simulink library "PV_lib"  (R2016b)
settings: Solver=ode45  StartTime=0.0  StopTime=10.0  RelTol=1e-3  EnableMultiTasking=on
undefined symbols (not defined in the file): C, D, DiscIntNeverNeededParam, f, I_ki, I_kp, Iac_max, Id_at_max, Iq_at_max, L, PLL_Ki, PLL_Kp, PLL_time_step, Roff, Tau, Td_es_min, Tds, Ts, Vdc_max
libraries: powerlib x42, simulink x16, cstextras x4, powerlib_extras x3, Batt_lib x1, powerlib_meascontrol x1
(part 1 of 2)
settings Model: Creator=re25624  LastModifiedBy=jlesage
settings DataIOCC: LimitDataPoints=on  SaveFormat=Array  SignalLoggingSaveFormat=ModelDataLogs
settings OptimizationCC: ExpressionDepthLimit=2147483647  LifeSpan=inf
settings DebuggingCC: UnderspecifiedInitializationDetection=Classic  MergeDetectMultiDrivingBlocksExec=none  SolverPrmCheckMsg=warning  FcnCallInpInsideContextMsg=warning  StateNameClashWarn=warning  SFUnexpectedBacktrackingDiag=warning  SFNoUnconditionalDefaultTransitionDiag=warning  SFExecutionAtInitializationDiag=none
settings HardwareCC: ProdBitPerPointer=32  ProdBitPerSizeT=32  ProdBitPerPtrDiffT=32  ProdLargestAtomicFloat=None  ProdIntDivRoundTo=Undefined  ProdEndianess=Unspecified  ProdWordSize=32  ProdHWDeviceType=32-bit Generic
settings ModelReferenceCC: PropagateSignalLabelsOutOfModel=off
settings GRTTargetCC: TargetLangStandard=C89/C90 (ANSI)  GeneratePreprocessorConditionals=Disable all  CombineOutputUpdateFcns=off  GRTInterface=on
settings ConfigComp: CovMetricSettings=dw  CovHtmlReporting=on  CovSaveCumulativeToWorkspaceVar=on  CovSaveSingleToWorkspaceVar=on  CovExternalEMLEnable=off

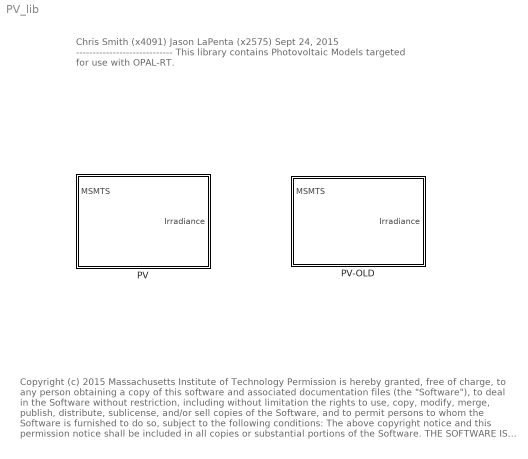
== system PV_lib ==
  note: Chris Smith (x4091)
      | Jason LaPenta (x2575)
      | Sept 24, 2015
      | -----------------------------
      | This library contains Photovoltaic Models
      | targeted for use with OPAL-RT.
  note: Copyright (c) 2015 Massachusetts Institute of Technology
      | Permission is hereby granted, free of charge, to any person obtaining a copy of this software and associated documentation files (the "Software"), to deal in the Software without restriction, including without limitation the rights to use, copy, modify, merge, publish, distribute, sublicense, and/or sell copies of the Software, and to permit persons to whom the Software is furnished to do so, subject to the following conditions:
      |
      | The above copyright notice and this permission notice shall be included in all copies or substantial portions of the Software.
      |
      | THE SOFTWARE IS PROVIDED "AS IS", WITHOUT WARRANTY OF ANY KIND, EXPRESS OR IMPLIED, INCLUDING BUT NOT LIMITED TO THE WARRANTIES OF MERCHANTABILITY, FITNESS FOR A PARTICULAR PURPOSE AND NONINFRINGEMENT. IN NO EVENT SHALL THE AUTHORS OR COPYRIGHT HOLDERS BE LIABLE FOR ANY CLAIM,
      | DAMAGES OR OTHER LIABILITY, WHETHER IN AN ACTION OF CONTRACT, TORT OR OTHERWISE, ARISING FROM, OUT OF OR IN CONNECTION WITH THE SOFTWARE OR THE USE OR OTHER DEALINGS IN THE SOFTWARE.
  PV : Subsystem  mask{max_power=4e6, VacRMS=1200, VacRMS_limit_pu=[1.1 0.9]}
      mask prompts: max_power "Peak Power (W)"; VacRMS "Grid Tie Line to Neutral Voltage (RMS)"; VacRMS_limit_pu "VacRMS Limit [Hi Low] (pu L-N)"
      mask TypeOptions max_power: PV System/max_power
      mask TypeOptions VacRMS: PV System/VacRMS
      mask TypeOptions VacRMS_limit_pu: PV System/VacRMS_limit_pu
  PV-OLD : Subsystem

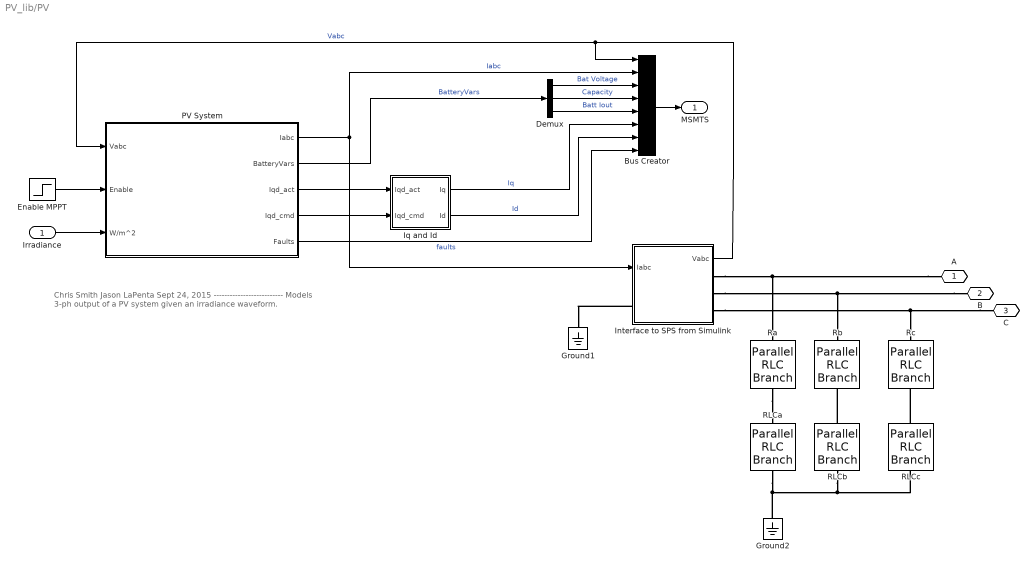
== system PV_lib/PV ==
  note: Chris Smith
      | Jason LaPenta
      | Sept 24, 2015
      | --------------------------
      | Models 3-ph output of a PV system
      | given an irradiance waveform.
  Irradiance : Inport
  Bus Creator : BusCreator  Inputs=8
  Demux : Demux  Outputs=3
  Enable MPPT : Step  Time=0.5  SampleTime=Ts
  Ground1 : powerlib/Elements/Ground  LConnTagsString=a
  Ground2 : powerlib/Elements/Ground  LConnTagsString=a
  Interface to SPS from Simulink : Subsystem
  Iq and Id : Subsystem
  PV System : Subsystem  mask(Battery Energy Storage System with AC inverter and Droop Control){max_power=max_power, VacRMS=VacRMS, Vdc_nom=3500, VacRMS_limit_pu=VacRMS_limit_pu}
      mask prompts: max_power "Peak Power (W)"; VacRMS "Grid Tie Line to Neutral Voltage (RMS)"; Vdc_nom "Nominal DC Battery Voltage"; VacRMS_limit_pu "VacRMS Limit [Hi Low] (pu L-N)"
      mask help: The block implements a battery energy storage system suitable for connecting to the grid. It responds to grid voltage changes by injecting current into the grid. The model is a non-switching average model.
      mask init:
      | %global_parameters
      | BES_init
      mask Help:
      | This block will likely need a filter and transformer on it's output in order to connect to a high power line.
      | 
      | A unit delay block  on the Iabc output can help remove algebraic loops with minimal impact on simulation results.
      | 
      | 
      | Block Parameters:
      | Peak Power- Maximum power the unit can transfer.
      | Capacity- Amount of energy in the battery.
      | Grid Tie Line to Neutral Voltage- RMS voltage for the grid tie interface.
      | Nominal DC Battery Voltage- Open circuit full charge voltage.
      | Real Power Droop Gain- Ratio of Watts to Hz for injecting power to the grid in response to frequency changes.
      | Reactive Power Droop Gain- Ratio of kVars to RMS volts for injecting reactive power to the grid.
      | Droop Filter Cut Off- Fastest frequency that will be responded to for injecting power to the grid.
      | 
      | 
      | Block Connections:
      | Vabc- Grid voltage for each of the three phases.
      | Enable- Set to zero for no power.  Set to 1 to enable energy tranfer.
      | Iabc- Grid current for each of the three phases.  Connect to your grid.  Positive is into the grid.
      | Battery_vars- A vector of battery voltage, capacity, and current out of the battery.
      | Iqd_cmd- Commanded q and d axis currents.
      | Iqd_act- Actual q and d axis currents.
      mask TypeOptions VacRMS_limit_pu: Grid Tied Inverter/VacRMS_limit_pu
  RLCa : powerlib/Elements/Parallel RLC Branch  LConnTagsString=a  RConnTagsString=__new0  BranchType=RLC  Resistance=1e6  Inductance=inf  SetiL0=off  InitialCurrent=0  Capacitance=10e-6  Setx0=off  InitialVoltage=0  Measurements=None
  RLCb : powerlib/Elements/Parallel RLC Branch  LConnTagsString=a  RConnTagsString=__new0  BranchType=RLC  Resistance=1e6  Inductance=inf  SetiL0=off  InitialCurrent=0  Capacitance=10e-6  Setx0=off  InitialVoltage=0  Measurements=None
  "RLCc " : powerlib/Elements/Parallel RLC Branch  LConnTagsString=a  RConnTagsString=__new0  BranchType=RLC  Resistance=1e6  Inductance=inf  SetiL0=off  InitialCurrent=0  Capacitance=10e-6  Setx0=off  InitialVoltage=0  Measurements=None
  Ra : powerlib/Elements/Parallel RLC Branch  LConnTagsString=a  RConnTagsString=__new0  BranchType=R  Resistance=10e-3  Inductance=inf  SetiL0=off  InitialCurrent=0  Capacitance=0  Setx0=off  InitialVoltage=0  Measurements=None
  Rb : powerlib/Elements/Parallel RLC Branch  LConnTagsString=a  RConnTagsString=__new0  BranchType=R  Resistance=10e-3  Inductance=inf  SetiL0=off  InitialCurrent=0  Capacitance=0  Setx0=off  InitialVoltage=0  Measurements=None
  Rc : powerlib/Elements/Parallel RLC Branch  LConnTagsString=a  RConnTagsString=__new0  BranchType=R  Resistance=10e-3  Inductance=inf  SetiL0=off  InitialCurrent=0  Capacitance=0  Setx0=off  InitialVoltage=0  Measurements=None
  A : PMIOPort  Port=1  Side=Right
  B : PMIOPort  Port=2  Side=Right
  C : PMIOPort  Port=3  Side=Right
  MSMTS : Outport
  wires:
  PV System/4(Iqd_cmd) -> Iq and Id/2(Iqd_cmd)
  PV System/5(Faults) -> Bus Creator/8  "faults"
  Enable MPPT/1 -> PV System/2(Enable)
  Bus Creator/1 -> MSMTS/1
  Iq and Id/2(Id) -> Bus Creator/7  "Id"
  PV System/1(Iabc) -> Bus Creator/2, Interface to SPS from Simulink/1(Iabc)  "Iabc"
  Iq and Id/1(Iq) -> Bus Creator/6  "Iq"
  PV System/3(Iqd_act) -> Iq and Id/1(Iqd_act)
  Demux/1 -> Bus Creator/3  "Bat Voltage"
  Demux/3 -> Bus Creator/5  "Batt Iout"
  Demux/2 -> Bus Creator/4  "Capacity"
  PV System/2(BatteryVars) -> Demux/1  "BatteryVars"
  Interface to SPS from Simulink/1(Vabc) -> Bus Creator/1, PV System/1(Vabc)  "Vabc"
  Irradiance/1 -> PV System/3(W/m^2)
  connections:
  Interface to SPS from Simulink/LConn1 -- Ground1/LConn1
  Ra/RConn1 -- RLCa/LConn1
  RLCb/LConn1 -- Rb/RConn1
  "RLCc "/LConn1 -- Rc/RConn1
  A/RConn1 -- Interface to SPS from Simulink/RConn1 -- Ra/LConn1
  C/RConn1 -- Interface to SPS from Simulink/RConn3 -- Rc/LConn1
  B/RConn1 -- Interface to SPS from Simulink/RConn2 -- Rb/LConn1
  "RLCc "/RConn1 -- RLCb/RConn1 -- RLCa/RConn1 -- Ground2/LConn1

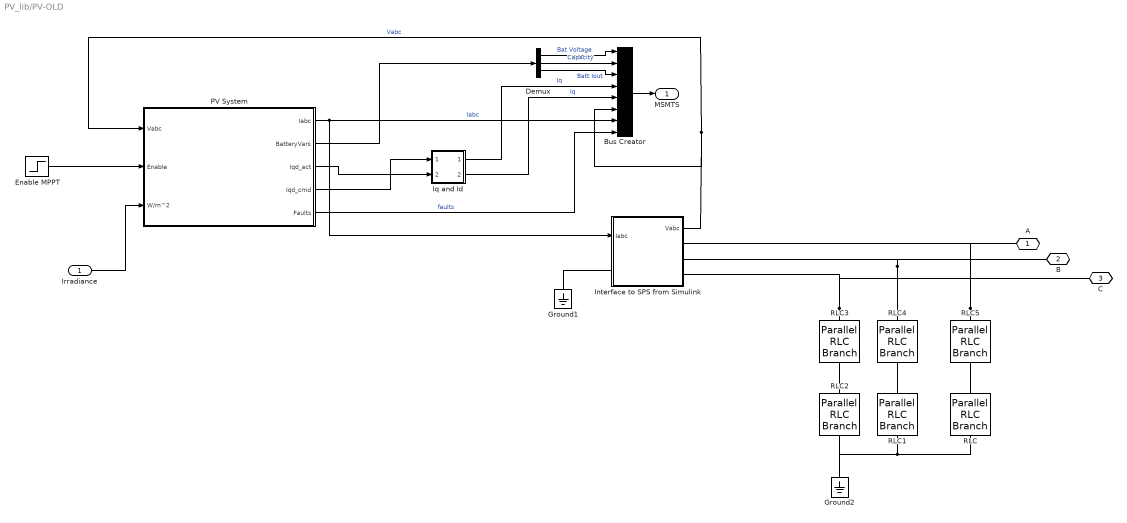
== system PV_lib/PV-OLD ==
  Irradiance : Inport
  Bus Creator : BusCreator  Inputs=8
  Demux : Demux  Outputs=3
  Enable MPPT : Step  Time=0.5  SampleTime=Ts
  Ground1 : powerlib/Elements/Ground  LConnTagsString=a
  Ground2 : powerlib/Elements/Ground  LConnTagsString=a
  Interface to SPS from Simulink : Subsystem
  Iq and Id : Subsystem
  PV System : Subsystem  mask(Battery Energy Storage System with AC inverter and Droop Control){max_power=4e6, VacRMS=1200, Vdc_nom=3500}
      mask prompts: max_power "Peak Power (W)"; VacRMS "Grid Tie Line to Neutral Voltage (RMS)"; Vdc_nom "Nominal DC Battery Voltage"
      mask help: The block implements a battery energy storage system suitable for connecting to the grid. It responds to grid voltage changes by injecting current into the grid. The model is a non-switching average model.
      mask init:
      | global_parameters
      | BES_init
      mask Help:
      | This block will likely need a filter and transformer on it's output in order to connect to a high power line.
      | 
      | A unit delay block  on the Iabc output can help remove algebraic loops with minimal impact on simulation results.
      | 
      | 
      | Block Parameters:
      | Peak Power- Maximum power the unit can transfer.
      | Capacity- Amount of energy in the battery.
      | Grid Tie Line to Neutral Voltage- RMS voltage for the grid tie interface.
      | Nominal DC Battery Voltage- Open circuit full charge voltage.
      | Real Power Droop Gain- Ratio of Watts to Hz for injecting power to the grid in response to frequency changes.
      | Reactive Power Droop Gain- Ratio of kVars to RMS volts for injecting reactive power to the grid.
      | Droop Filter Cut Off- Fastest frequency that will be responded to for injecting power to the grid.
      | 
      | 
      | Block Connections:
      | Vabc- Grid voltage for each of the three phases.
      | Enable- Set to zero for no power.  Set to 1 to enable energy tranfer.
      | Iabc- Grid current for each of the three phases.  Connect to your grid.  Positive is into the grid.
      | Battery_vars- A vector of battery voltage, capacity, and current out of the battery.
      | Iqd_cmd- Commanded q and d axis currents.
      | Iqd_act- Actual q and d axis currents.
  "RLC " : powerlib/Elements/Parallel RLC Branch  LConnTagsString=a  RConnTagsString=__new0  BranchType=RLC  Resistance=1e6  Inductance=inf  SetiL0=off  InitialCurrent=0  Capacitance=10e-6  Setx0=off  InitialVoltage=0  Measurements=None
  RLC1 : powerlib/Elements/Parallel RLC Branch  LConnTagsString=a  RConnTagsString=__new0  BranchType=RLC  Resistance=1e6  Inductance=inf  SetiL0=off  InitialCurrent=0  Capacitance=10e-6  Setx0=off  InitialVoltage=0  Measurements=None
  RLC2 : powerlib/Elements/Parallel RLC Branch  LConnTagsString=a  RConnTagsString=__new0  BranchType=RLC  Resistance=1e6  Inductance=inf  SetiL0=off  InitialCurrent=0  Capacitance=10e-6  Setx0=off  InitialVoltage=0  Measurements=None
  RLC3 : powerlib/Elements/Parallel RLC Branch  LConnTagsString=a  RConnTagsString=__new0  BranchType=R  Resistance=10e-3  Inductance=inf  SetiL0=off  InitialCurrent=0  Capacitance=0  Setx0=off  InitialVoltage=0  Measurements=None
  RLC4 : powerlib/Elements/Parallel RLC Branch  LConnTagsString=a  RConnTagsString=__new0  BranchType=R  Resistance=10e-3  Inductance=inf  SetiL0=off  InitialCurrent=0  Capacitance=0  Setx0=off  InitialVoltage=0  Measurements=None
  RLC5 : powerlib/Elements/Parallel RLC Branch  LConnTagsString=a  RConnTagsString=__new0  BranchType=R  Resistance=10e-3  Inductance=inf  SetiL0=off  InitialCurrent=0  Capacitance=0  Setx0=off  InitialVoltage=0  Measurements=None
  A : PMIOPort  Port=1  Side=Right
  B : PMIOPort  Port=2  Side=Right
  C : PMIOPort  Port=3  Side=Right
  MSMTS : Outport
  wires:
  PV System/4(Iqd_cmd) -> Iq and Id/1(In1)
  PV System/5(Faults) -> Bus Creator/8  "faults"
  Enable MPPT/1 -> PV System/2(Enable)
  Bus Creator/1 -> MSMTS/1
  Iq and Id/2(Out2) -> Bus Creator/5  "Iq"
  PV System/1(Iabc) -> Interface to SPS from Simulink/1(Iabc), Bus Creator/7  "Iabc"
  Iq and Id/1(Out1) -> Bus Creator/4  "Iq"
  PV System/3(Iqd_act) -> Iq and Id/2(In2)
  Demux/1 -> Bus Creator/1  "Bat Voltage"
  Demux/3 -> Bus Creator/3  "Batt Iout"
  Demux/2 -> Bus Creator/2  "Capacity"
  PV System/2(BatteryVars) -> Demux/1
  Interface to SPS from Simulink/1(Vabc) -> PV System/1(Vabc), Bus Creator/6  "Vabc"
  Irradiance/1 -> PV System/3(W/m^2)
  connections:
  "RLC "/LConn1 -- RLC5/RConn1
  RLC1/LConn1 -- RLC4/RConn1
  RLC3/RConn1 -- RLC2/LConn1
  RLC5/LConn1 -- A/RConn1 -- Interface to SPS from Simulink/RConn1
  RLC3/LConn1 -- C/RConn1 -- Interface to SPS from Simulink/RConn3
  Interface to SPS from Simulink/RConn2 -- B/RConn1 -- RLC4/LConn1
  RLC1/RConn1 -- "RLC "/RConn1 -- RLC2/RConn1 -- Ground2/LConn1
  Interface to SPS from Simulink/LConn1 -- Ground1/LConn1

== system PV_lib/PV/Interface to SPS from Simulink ==
  Iabc : Inport
  Demux4 : Demux  Outputs=3
  Gain : Gain  Gain=-1
  Ia : powerlib/Electrical Sources/Controlled Current Source  Initialize=on  Source_Type=AC  Amplitude=0  Phase=0  Frequency=0  Measurements=None
  Ib : powerlib/Electrical Sources/Controlled Current Source  Initialize=on  Source_Type=AC  Amplitude=0  Phase=0  Frequency=0  Measurements=None
  Ic : powerlib/Electrical Sources/Controlled Current Source  Initialize=on  Source_Type=AC  Amplitude=0  Phase=0  Frequency=0  Measurements=None
  Mux2 : Mux  Inputs=3
  Va : powerlib/Measurements/Voltage Measurement  PhasorSimulation=off  OutputType=Complex  PSBequivalent=0
  Vb : powerlib/Measurements/Voltage Measurement  PhasorSimulation=off  OutputType=Complex  PSBequivalent=0
  Vc : powerlib/Measurements/Voltage Measurement  PhasorSimulation=off  OutputType=Complex  PSBequivalent=0
  Phase_A : PMIOPort  Port=1  Side=Right
  Phase_B : PMIOPort  Port=2  Side=Right
  Phase_C : PMIOPort  Port=3  Side=Right
  Ground : PMIOPort  Port=4  Side=Left
  Vabc : Outport
  wires:
  Gain/1 -> Demux4/1
  Va/1 -> Mux2/1
  Mux2/1 -> Vabc/1
  Iabc/1 -> Gain/1
  Demux4/3 -> Ic/1
  Demux4/2 -> Ib/1
  Demux4/1 -> Ia/1
  Vb/1 -> Mux2/2
  Vc/1 -> Mux2/3
  connections:
  Phase_B/RConn1 -- Ib/RConn1 -- Vb/LConn1
  Ground/RConn1 -- Vc/LConn2 -- Va/LConn2 -- Vb/LConn2 -- Ib/LConn1 -- Ia/LConn1 -- Ic/LConn1
  Phase_C/RConn1 -- Ic/RConn1 -- Vc/LConn1
  Ia/RConn1 -- Va/LConn1 -- Phase_A/RConn1

== system PV_lib/PV/Iq and Id ==
  Iqd_act : Inport
  Iqd_cmd : Inport  Port=2
  Demux1 : Demux  Outputs=2
  Demux2 : Demux  Outputs=2
  Mux : Mux  Inputs=2
  Mux1 : Mux  Inputs=2
  Iq : Outport
  Id : Outport  Port=2
  wires:
  Demux1/2 -> Mux1/1  "Id_cmd"
  Demux2/1 -> Mux/2  "Iq_act"
  Demux1/1 -> Mux/1  "Iq_cmd"
  Demux2/2 -> Mux1/2  "Id_act"
  Iqd_cmd/1 -> Demux1/1
  Iqd_act/1 -> Demux2/1
  Mux/1 -> Iq/1
  Mux1/1 -> Id/1

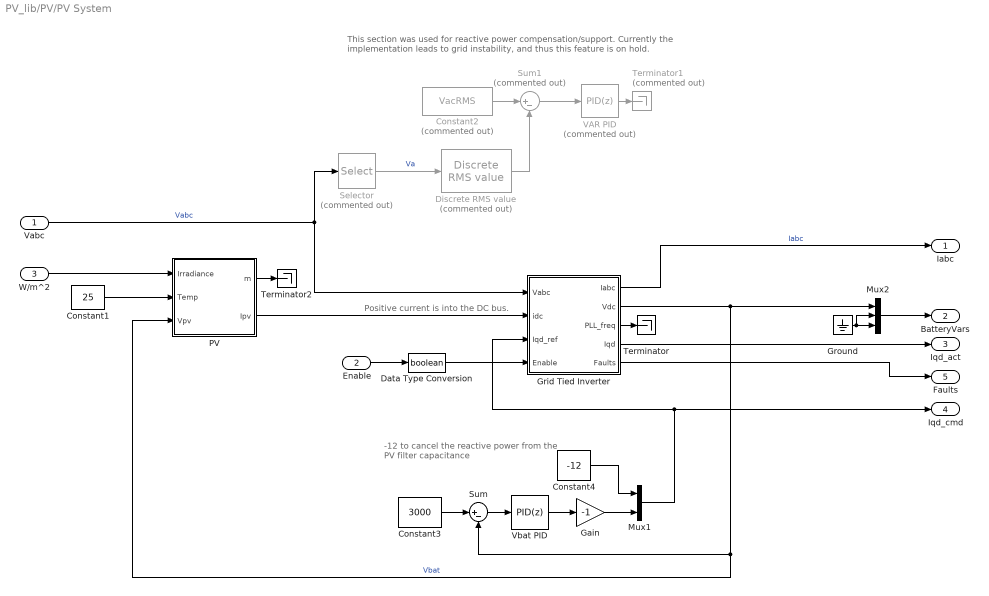
== system PV_lib/PV/PV System ==
  note: Positive current is into the DC bus.
  note: This section was used for reactive power compensation/support.
      | Currently the implementation leads to grid instability, and thus
      | this feature is on hold.
  note: -12 to cancel the reactive power
      | from the PV filter capacitance
  Vabc : Inport
  Enable : Inport  Port=2  OutDataTypeStr=double
  W/m^2 : Inport  Port=3
  Constant1 : Constant  Value=25
  Constant2 : Constant  Commented=on  Value=VacRMS
  Constant3 : Constant  Value=3000
  Constant4 : Constant  Value=-12
  Data Type Conversion : DataTypeConversion  OutDataTypeStr=boolean
  Discrete RMS value : powerlib_extras/Discrete Measurements/Discrete  RMS value  Commented=on  Freq=60  Mag_Init=1200  Ts=Ts
  Gain : Gain  Gain=-1
  Grid Tied Inverter : Subsystem  mask{VacRMS_limit_pu=VacRMS_limit_pu}
      mask prompts: VacRMS_limit_pu "VacRMS Limit [Hi Low] (pu L-N)"
  Ground : Ground
  Mux1 : Mux  Inputs=2
  Mux2 : Mux  Inputs=3
  PV : Subsystem  mask{Ncell=60, Nser=102, Npar=158, Voc_Tref=38, Isc_Tref=8.9, Eg=1.12, dVdI_Voc=-0.32, K0=0.05, Rs=0.349, Rsh=111.55, IL=8.944, Vm=30.5, Im=8.03, PlotVI_module=off, PlotVI_array=off}
      mask prompts: Ncell "Number of cells per module"; Nser "Number of series-connected module per string"; Npar "Numer of parallel strings"; Voc_Tref "Open circuit voltage Voc (V)"; Isc_Tref "Short circuit current Isc (A)"; Eg "Band gap energy of crystalline silicon (eV)"; dVdI_Voc "Temperature coefficient of Voc (%/C)"; K0 "Temperature coefficient of Isc (%/C)"; Rs "Series resistance Rs (Ohms)"; Rsh "Shunt resistance Rsh (Ohms)"; IL "Light-generated current IL (A)"; Vm "Maximum Power Point Voltage Vmpp (V)"; Im "Maximum Powe Point Current Impp (A)"; PlotVI_module "Display  I-V and  P-V characteritics of one module"; PlotVI_array "Display  I-V and  P-V characteritics of array"
      mask init:
      | BlockName=gcb;
      | 
      | 
      | q = 1.6022e-19; % electron charge
      | k = 1.3806e-23; % Boltzman constant
      | n = 1.55; % diode quality factor
      | Tref_K = 273.15+25; % 25C to K
      | Gnom = 1000; % nominal irradiation in W/m^2
      | VT_ref = Ncell*n*k*Tref_K/q; 
      | I0_Tref = Isc_Tref/(exp(Voc_Tref/VT_ref)-1);
      | % Xv = I0_Tref*q*exp(Voc_Tref/VT_ref)/n/k/Tref_K;
      | % Rs = -dVdI_Voc-1/Xv; 
      | 
      | %% Plot I-V & P-V characteristics of one module
      | %==============================================
      | if PlotVI_module | PlotVI_array
      |     assignin('base','Voc_Tref',Voc_Tref);
      |     assignin('base','Isc_Tref',Isc_Tref);
      |     assignin('base','Rs',Rs);
      |     assignin('base','Rsh',Rsh);
      |     assignin('base','I0_Tref',I0_Tref);
      |     assignin('base','VT_ref',VT_ref);
      |      
      |     if PlotVI_module, 
      |         F1 = figure('Name','I-V characteristics of one module at 25 deg.C');
      |         F2 = figure('Name','P-V characteristics of one module at 25 deg.C');
      |     end
      |     if PlotVI_array ,
      |         F3 = figure('Name','I-V characteristics of array at 25 deg.C'); 
      |         F4 = figure('Name','P-V characteristics of array at 25 deg.C'); 
      |     end
      |     load_system('PV_param_plot_model');
      |     
      |     for ksun = 1:-0.2:0.2
      |         assignin('base','IL',IL*ksun)
      |         sim('PV_param_plot_model');
      |         n = find(I_PV >= 0);
      |         I_PV = I_PV(n);
      |         V_PV = V_PV(n);
      |         P_PV = V_PV.*I_PV;
      |         
      |         if PlotVI_module
      |             figure(F1);
      |             if ksun == 1
      |                 
      |                 plot(V_PV,I_PV,'b')
      |                % plot(V_PV,I_PV,'b',[0  Vm Voc_Tref], [Isc_Tref Im 0],'ro')
      |                 text(Voc_Tref/15,Isc_Tref*1.1,'1 kW/m^2')
      |                 hold on
      |                 grid
      |             else
      |                 plot(V_PV,I_PV,'--m')
      |                 text(Voc_Tref/15, Isc_Tref*(ksun+0.1) , sprintf('%g kW/m^2',ksun))
      |             end
      | 
      |             figure(F2); 
      |             if ksun == 1
      |                 
      |                 plot(V_PV,I_PV,'b')
      |                 %plot(V_PV,P_PV,'b',[0  Vm Voc_Tref], [0 Im*Vm 0],'ro')
      |                 text(Vm*1.02,Vm*Im,'1 kW/m^2')
      |                 hold on
      |                 grid
      |             else
      |                 n = find(P_PV == max(P_PV));
      |                 % plot(V_PV,P_PV,'--m', V_PV(n) , P_PV(n),'mo')
      |                 plot(V_PV,P_PV,'--m')
      |                 text(Vm*1.02, Vm*Im*ksun, sprintf('%g kW/m^2',ksun))
      |             end
      |             figure(F1); 
      |             ylabel('Current (A)')
      |             xlabel('Voltage (V)')
      |             axis_xy = axis;
      |             axis_xy(4) = Isc_Tref*1.2;
      |             axis(axis_xy);
      |             
      |             figure(F2);
      |             ylabel('Power (W)')
      |             xlabel('Voltage (V)')
      |             axis_xy = axis;
      |             axis_xy(4) = Vm*Im*1.2;
      |             axis(axis_xy);
      |                   
      |             set_param(BlockName,'PlotVI_module', 'off')
      |         end
      |         
      |         if PlotVI_array
      |             figure(F3);
      |             if ksun == 1
      |                 plot(V_PV*Nser,I_PV*Npar,'b')
      |                 % plot(V_PV*Nser,I_PV*Npar,'b',[0  Vm Voc_Tref]*Nser, [Isc_Tref Im 0]*Npar,'ro')
      |                 text(Voc_Tref/15*Nser,Isc_Tref*1.1*Npar,'1 kW/m^2')
      |                 hold on
      |                 grid
      |             else
      |                 plot(V_PV*Nser,I_PV*Npar,'--m')
      |                 text(Voc_Tref*Nser/15, Isc_Tref*Npar*(ksun+0.1) , sprintf('%g kW/m^2',ksun))
      |             end
      |            
      | 
      |             figure(F4);
      |             if ksun == 1
      |                 plot(V_PV*Nser,P_PV*Nser*Npar,'b')
      |                 % plot(V_PV*Nser,P_PV*Nser*Npar,'b',[0  Vm Voc_Tref]*Nser, [0 Im*Vm 0]*Nser*Npar,'ro')
      |                 text(Vm*Nser*1.02,Vm*Im*Nser*Npar,'1 kW/m^2')
      |                 hold on
      |                 grid
      |             else
      |                 n = find(P_PV == max(P_PV));
      |                 plot(V_PV*Nser,P_PV*Nser*Npar,'--m')
      |                 % plot(V_PV*Nser,P_PV*Nser*Npar,'--m', V_PV(n)*Nser , P_PV(n)*Nser*Npar,'mo')
      |                 text(Vm*Nser*1.02, Vm*Im*Nser*Npar*ksun, sprintf('%g kW/m^2',ksun))
      |             end 
      |             figure(F3);
      |             ylabel('Current (A)')
      |             xlabel('Voltage (V)')
      |             axis_xy = axis;
      |             axis_xy(4) = Isc_Tref*Npar*1.2;
      |             axis(axis_xy);
      |             
      |             figure(F4);
      |             ylabel('Power (W)')
      |             xlabel('Voltage (V)')
      |             xis_xy = axis;
      |             axis_xy(4) = Vm*Im*Nser*Npar*1.2;
      |             axis(axis_xy);
      |             
      |             set_param(BlockName,'PlotVI_array', 'off')
      |         end
      |         
      |     end  
      | end
  Selector : Selector  Commented=on  InputPortWidth=3  IndexOptions=Index vector (dialog)  Indices=[1]  OutputSizes=1
  Sum : Sum  Inputs=|+-
  Sum1 : Sum  Commented=on  Inputs=|+-
  Terminator : Terminator
  Terminator1 : Terminator  Commented=on
  Terminator2 : Terminator
  VAR PID : simulink/Continuous/PID Controller  Commented=on  Controller=PID  TimeDomain=Discrete-time  SampleTime=Ts  IntegratorMethod=Forward Euler  FilterMethod=Forward Euler  Form=Parallel  UseFilter=on  ControllerParametersSource=internal  P=4  I=3  D=0  N=100  InitialConditionSource=internal  InitialConditionForIntegrator=0  InitialConditionForFilter=0  ExternalReset=none  LimitOutput=on  UpperSaturationLimit=2000  LowerSaturationLimit=-2000  LinearizeAsGain=off  AntiWindupMode=clamping  Kb=1  TrackingMode=off  Kt=1  PParamMin=[]  PParamMax=[]  IParamMin=[]  IParamMax=[]  DParamMin=[]  DParamMax=[]  NParamMin=[]  NParamMax=[]  KbParamMin=[]  KbParamMax=[]  KtParamMin=[]  KtParamMax=[]  POutMin=[]  POutMax=[]  IOutMin=[]  IOutMax=[]  DOutMin=[]  DOutMax=[]  NOutMin=[]  NOutMax=[]  KbOutMin=[]  KbOutMax=[]  KtOutMin=[]  KtOutMax=[]  IntegratorOutMin=[]  IntegratorOutMax=[]  FilterOutMin=[]  FilterOutMax=[]  SumOutMin=[]  SumOutMax=[]  SumI1OutMin=[]  SumI1OutMax=[]  SumI2OutMin=[]  SumI2OutMax=[]  SumI3OutMin=[]  SumI3OutMax=[]  SumDOutMin=[]  SumDOutMax=[]  SaturationOutMin=[]  SaturationOutMax=[]  IntegratorContinuousStateAttributes=''  IntegratorStateMustResolveToSignalObject=off  IntegratorRTWStateStorageClass=Auto  FilterContinuousStateAttributes=''  FilterStateMustResolveToSignalObject=off  FilterRTWStateStorageClass=Auto  DifferentiatorICPrevScaledInput=0  DifferentiatorOutMin=[]  DifferentiatorOutMax=[]
  Vbat PID : simulink/Continuous/PID Controller  Controller=PID  TimeDomain=Discrete-time  SampleTime=Ts  IntegratorMethod=Forward Euler  FilterMethod=Forward Euler  Form=Parallel  UseFilter=on  ControllerParametersSource=internal  P=4  I=3  D=0  N=100  InitialConditionSource=internal  InitialConditionForIntegrator=0  InitialConditionForFilter=0  ExternalReset=none  LimitOutput=on  UpperSaturationLimit=2000  LowerSaturationLimit=-2000  LinearizeAsGain=off  AntiWindupMode=clamping  Kb=1  TrackingMode=off  Kt=1  PParamMin=[]  PParamMax=[]  IParamMin=[]  IParamMax=[]  DParamMin=[]  DParamMax=[]  NParamMin=[]  NParamMax=[]  KbParamMin=[]  KbParamMax=[]  KtParamMin=[]  KtParamMax=[]  POutMin=[]  POutMax=[]  IOutMin=[]  IOutMax=[]  DOutMin=[]  DOutMax=[]  NOutMin=[]  NOutMax=[]  KbOutMin=[]  KbOutMax=[]  KtOutMin=[]  KtOutMax=[]  IntegratorOutMin=[]  IntegratorOutMax=[]  FilterOutMin=[]  FilterOutMax=[]  SumOutMin=[]  SumOutMax=[]  SumI1OutMin=[]  SumI1OutMax=[]  SumI2OutMin=[]  SumI2OutMax=[]  SumI3OutMin=[]  SumI3OutMax=[]  SumDOutMin=[]  SumDOutMax=[]  SaturationOutMin=[]  SaturationOutMax=[]  IntegratorContinuousStateAttributes=''  IntegratorStateMustResolveToSignalObject=off  IntegratorRTWStateStorageClass=Auto  FilterContinuousStateAttributes=''  FilterStateMustResolveToSignalObject=off  FilterRTWStateStorageClass=Auto  DifferentiatorICPrevScaledInput=0  DifferentiatorOutMin=[]  DifferentiatorOutMax=[]
  Iabc : Outport
  BatteryVars : Outport  Port=2
  Iqd_act : Outport  Port=3
  Iqd_cmd : Outport  Port=4
  Faults : Outport  Port=5
  wires:
  Grid Tied Inverter/5(Faults) -> Faults/1
  Mux1/1 -> Grid Tied Inverter/3(Iqd_ref), Iqd_cmd/1
  Constant4/1 -> Mux1/1
  Selector/1 -> Discrete RMS value/1  "Va"
  Discrete RMS value/1 -> Sum1/2
  Constant2/1 -> Sum1/1
  Sum1/1 -> VAR PID/1
  Gain/1 -> Mux1/2
  Constant3/1 -> Sum/1
  Vbat PID/1 -> Gain/1
  Sum/1 -> Vbat PID/1
  PV/2(Ipv) -> Grid Tied Inverter/2(idc)
  Constant1/1 -> PV/2(Temp)
  W/m^2/1 -> PV/1(Irradiance)
  Vabc/1 -> Grid Tied Inverter/1(Vabc), Selector/1  "Vabc"
  Grid Tied Inverter/2(Vdc) -> PV/3(Vpv), Sum/2, Mux2/1  "Vbat"
  Grid Tied Inverter/1(Iabc) -> Iabc/1  "Iabc"
  Grid Tied Inverter/4(Iqd) -> Iqd_act/1
  Enable/1 -> Data Type Conversion/1
  Data Type Conversion/1 -> Grid Tied Inverter/4(Enable)
  Mux2/1 -> BatteryVars/1
  Grid Tied Inverter/3(PLL_freq) -> Terminator/1
  VAR PID/1 -> Terminator1/1
  Ground/1 -> Mux2/2, Mux2/3
  PV/1(m) -> Terminator2/1

== system PV_lib/PV-OLD/Interface to SPS from Simulink ==
  Iabc : Inport
  Controlled Current Source3 : powerlib/Electrical Sources/Controlled Current Source  Initialize=on  Source_Type=AC  Amplitude=0  Phase=0  Frequency=0  Measurements=None
  Controlled Current Source4 : powerlib/Electrical Sources/Controlled Current Source  Initialize=on  Source_Type=AC  Amplitude=0  Phase=0  Frequency=0  Measurements=None
  Controlled Current Source5 : powerlib/Electrical Sources/Controlled Current Source  Initialize=on  Source_Type=AC  Amplitude=0  Phase=0  Frequency=0  Measurements=None
  Demux4 : Demux  Outputs=3
  Gain : Gain  Gain=-1
  Mux2 : Mux  Inputs=3
  Voltage Measurement3 : powerlib/Measurements/Voltage Measurement  PhasorSimulation=off  OutputType=Complex  PSBequivalent=0
  Voltage Measurement4 : powerlib/Measurements/Voltage Measurement  PhasorSimulation=off  OutputType=Complex  PSBequivalent=0
  Voltage Measurement5 : powerlib/Measurements/Voltage Measurement  PhasorSimulation=off  OutputType=Complex  PSBequivalent=0
  Phase_A : PMIOPort  Port=1  Side=Right
  Phase_B : PMIOPort  Port=2  Side=Right
  Phase_C : PMIOPort  Port=3  Side=Right
  Ground : PMIOPort  Port=4  Side=Left
  Vabc : Outport
  wires:
  Voltage Measurement5/1 -> Mux2/3
  Voltage Measurement4/1 -> Mux2/2
  Demux4/1 -> Controlled Current Source3/1
  Demux4/2 -> Controlled Current Source4/1
  Demux4/3 -> Controlled Current Source5/1
  Iabc/1 -> Gain/1
  Mux2/1 -> Vabc/1
  Voltage Measurement3/1 -> Mux2/1
  Gain/1 -> Demux4/1
  connections:
  Voltage Measurement5/LConn1 -- Controlled Current Source5/RConn1 -- Phase_C/RConn1
  Voltage Measurement3/LConn1 -- Controlled Current Source3/RConn1 -- Phase_A/RConn1
  Controlled Current Source5/LConn1 -- Controlled Current Source3/LConn1 -- Controlled Current Source4/LConn1 -- Voltage Measurement4/LConn2 -- Voltage Measurement3/LConn2 -- Voltage Measurement5/LConn2 -- Ground/RConn1
  Voltage Measurement4/LConn1 -- Controlled Current Source4/RConn1 -- Phase_B/RConn1

== system PV_lib/PV-OLD/Iq and Id ==
  In1 : Inport
  In2 : Inport  Port=2
  Demux1 : Demux  Outputs=2
  Demux2 : Demux  Outputs=2
  Mux : Mux  Inputs=2
  Mux1 : Mux  Inputs=2
  Out1 : Outport
  Out2 : Outport  Port=2
  wires:
  Mux1/1 -> Out2/1
  Mux/1 -> Out1/1
  In2/1 -> Demux2/1
  In1/1 -> Demux1/1
  Demux2/2 -> Mux1/2  "Id_act"
  Demux1/1 -> Mux/1  "Iq_cmd"
  Demux2/1 -> Mux/2  "Iq_act"
  Demux1/2 -> Mux1/1  "Id_cmd"

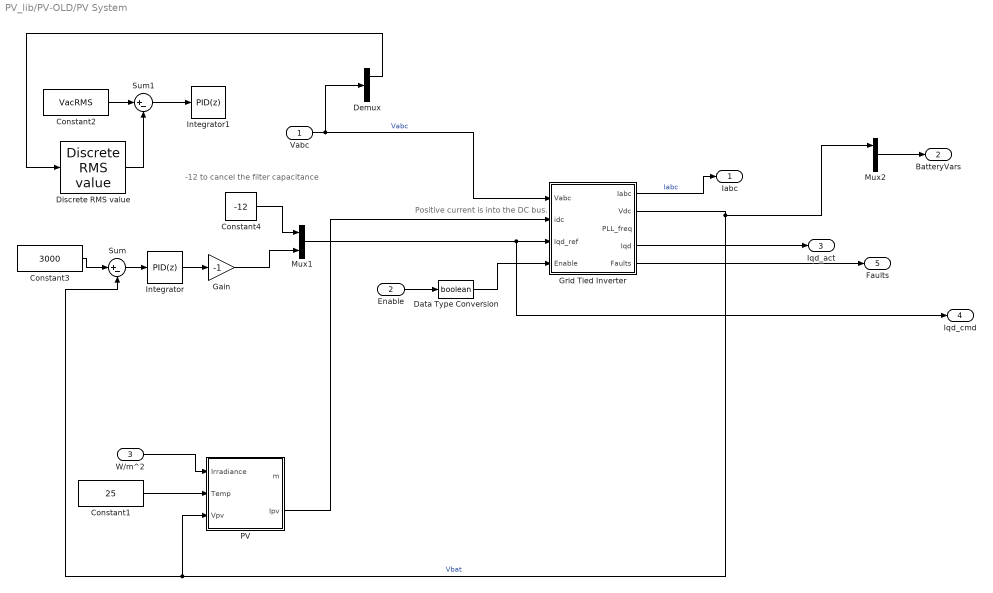
== system PV_lib/PV-OLD/PV System ==
  note: Positive current is into the DC bus.
  note: -12 to cancel the filter capacitance
  Vabc : Inport
  Enable : Inport  Port=2  OutDataTypeStr=double
  W/m^2 : Inport  Port=3
  Constant1 : Constant  Value=25
  Constant2 : Constant  Value=VacRMS
  Constant3 : Constant  Value=3000
  Constant4 : Constant  Value=-12
  Data Type Conversion : DataTypeConversion  OutDataTypeStr=boolean
  Demux : Demux  Outputs=3
  Discrete RMS value : powerlib_extras/Discrete Measurements/Discrete  RMS value  Freq=60  Mag_Init=1200  Ts=Ts
  Gain : Gain  Gain=-1
  Grid Tied Inverter : Subsystem
  Integrator : simulink/Continuous/PID Controller  Controller=PID  TimeDomain=Discrete-time  SampleTime=Ts  IntegratorMethod=Forward Euler  FilterMethod=Forward Euler  Form=Parallel  UseFilter=on  ControllerParametersSource=internal  P=4  I=3  D=0  N=100  InitialConditionSource=internal  InitialConditionForIntegrator=0  InitialConditionForFilter=0  ExternalReset=none  LimitOutput=on  UpperSaturationLimit=2000  LowerSaturationLimit=-2000  LinearizeAsGain=off  AntiWindupMode=clamping  Kb=1  TrackingMode=off  Kt=1  PParamMin=[]  PParamMax=[]  IParamMin=[]  IParamMax=[]  DParamMin=[]  DParamMax=[]  NParamMin=[]  NParamMax=[]  KbParamMin=[]  KbParamMax=[]  KtParamMin=[]  KtParamMax=[]  POutMin=[]  POutMax=[]  IOutMin=[]  IOutMax=[]  DOutMin=[]  DOutMax=[]  NOutMin=[]  NOutMax=[]  KbOutMin=[]  KbOutMax=[]  KtOutMin=[]  KtOutMax=[]  IntegratorOutMin=[]  IntegratorOutMax=[]  FilterOutMin=[]  FilterOutMax=[]  SumOutMin=[]  SumOutMax=[]  SumI1OutMin=[]  SumI1OutMax=[]  SumI2OutMin=[]  SumI2OutMax=[]  SumI3OutMin=[]  SumI3OutMax=[]  SumDOutMin=[]  SumDOutMax=[]  SaturationOutMin=[]  SaturationOutMax=[]  IntegratorContinuousStateAttributes=''  IntegratorStateMustResolveToSignalObject=off  IntegratorRTWStateStorageClass=Auto  FilterContinuousStateAttributes=''  FilterStateMustResolveToSignalObject=off  FilterRTWStateStorageClass=Auto  DifferentiatorICPrevScaledInput=0  DifferentiatorOutMin=[]  DifferentiatorOutMax=[]
  Integrator1 : simulink/Continuous/PID Controller  Controller=PID  TimeDomain=Discrete-time  SampleTime=Ts  IntegratorMethod=Forward Euler  FilterMethod=Forward Euler  Form=Parallel  UseFilter=on  ControllerParametersSource=internal  P=4  I=3  D=0  N=100  InitialConditionSource=internal  InitialConditionForIntegrator=0  InitialConditionForFilter=0  ExternalReset=none  LimitOutput=on  UpperSaturationLimit=2000  LowerSaturationLimit=-2000  LinearizeAsGain=off  AntiWindupMode=clamping  Kb=1  TrackingMode=off  Kt=1  PParamMin=[]  PParamMax=[]  IParamMin=[]  IParamMax=[]  DParamMin=[]  DParamMax=[]  NParamMin=[]  NParamMax=[]  KbParamMin=[]  KbParamMax=[]  KtParamMin=[]  KtParamMax=[]  POutMin=[]  POutMax=[]  IOutMin=[]  IOutMax=[]  DOutMin=[]  DOutMax=[]  NOutMin=[]  NOutMax=[]  KbOutMin=[]  KbOutMax=[]  KtOutMin=[]  KtOutMax=[]  IntegratorOutMin=[]  IntegratorOutMax=[]  FilterOutMin=[]  FilterOutMax=[]  SumOutMin=[]  SumOutMax=[]  SumI1OutMin=[]  SumI1OutMax=[]  SumI2OutMin=[]  SumI2OutMax=[]  SumI3OutMin=[]  SumI3OutMax=[]  SumDOutMin=[]  SumDOutMax=[]  SaturationOutMin=[]  SaturationOutMax=[]  IntegratorContinuousStateAttributes=''  IntegratorStateMustResolveToSignalObject=off  IntegratorRTWStateStorageClass=Auto  FilterContinuousStateAttributes=''  FilterStateMustResolveToSignalObject=off  FilterRTWStateStorageClass=Auto  DifferentiatorICPrevScaledInput=0  DifferentiatorOutMin=[]  DifferentiatorOutMax=[]
  Mux1 : Mux  Inputs=2
  Mux2 : Mux  Inputs=3
  PV : Subsystem  mask{Ncell=60, Nser=102, Npar=158, Voc_Tref=38, Isc_Tref=8.9, Eg=1.12, dVdI_Voc=-0.32, K0=0.05, Rs=0.349, Rsh=111.55, IL=8.944, Vm=30.5, Im=8.03, PlotVI_module=off, PlotVI_array=off}
      mask prompts: Ncell "Number of cells per module"; Nser "Number of series-connected module per string"; Npar "Numer of parallel strings"; Voc_Tref "Open circuit voltage Voc (V)"; Isc_Tref "Short circuit current Isc (A)"; Eg "Band gap energy of crystalline silicon (eV)"; dVdI_Voc "Temperature coefficient of Voc (%/C)"; K0 "Temperature coefficient of Isc (%/C)"; Rs "Series resistance Rs (Ohms)"; Rsh "Shunt resistance Rsh (Ohms)"; IL "Light-generated current IL (A)"; Vm "Maximum Power Point Voltage Vmpp (V)"; Im "Maximum Powe Point Current Impp (A)"; PlotVI_module "Display  I-V and  P-V characteritics of one module"; PlotVI_array "Display  I-V and  P-V characteritics of array"
      mask init: same as PV_lib/PV/PV System/PV
  Sum : Sum  Inputs=|+-
  Sum1 : Sum  Inputs=|+-
  Iabc : Outport
  BatteryVars : Outport  Port=2
  Iqd_act : Outport  Port=3
  Iqd_cmd : Outport  Port=4
  Faults : Outport  Port=5
  wires:
  Mux2/1 -> BatteryVars/1
  Data Type Conversion/1 -> Grid Tied Inverter/4(Enable)
  Enable/1 -> Data Type Conversion/1
  Grid Tied Inverter/4(Iqd) -> Iqd_act/1
  Grid Tied Inverter/1(Iabc) -> Iabc/1  "Iabc"
  Grid Tied Inverter/2(Vdc) -> Mux2/1, PV/3(Vpv), Sum/2  "Vbat"
  Vabc/1 -> Grid Tied Inverter/1(Vabc), Demux/1  "Vabc"
  W/m^2/1 -> PV/1(Irradiance)
  Constant1/1 -> PV/2(Temp)
  PV/2(Ipv) -> Grid Tied Inverter/2(idc)
  Mux1/1 -> Grid Tied Inverter/3(Iqd_ref), Iqd_cmd/1
  Sum/1 -> Integrator/1
  Integrator/1 -> Gain/1
  Constant3/1 -> Sum/1
  Gain/1 -> Mux1/2
  Sum1/1 -> Integrator1/1
  Constant2/1 -> Sum1/1
  Discrete RMS value/1 -> Sum1/2
  Demux/1 -> Discrete RMS value/1
  Grid Tied Inverter/5(Faults) -> Faults/1
  Constant4/1 -> Mux1/1

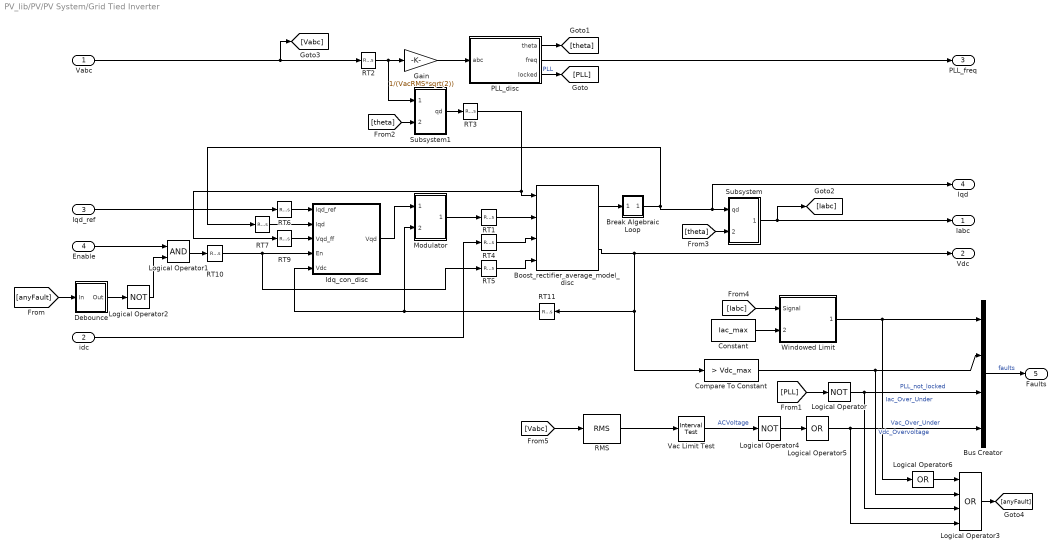
== system PV_lib/PV/PV System/Grid Tied Inverter ==
  Vabc : Inport
  idc : Inport  Port=2
  Iqd_ref : Inport  Port=3
  Enable : Inport  Port=4
  Boost_rectifier_average_model_disc : Batt_lib/HIL_BATT/Batt/Grid Tied Inverter/Boost_rectifier_average_model_disc  C=C  L=L  Roff=Roff  Vdc_nom=Vdc_nom
  Break Algebraic Loop : Subsystem  mask{Tau=Tau, Ts=Ts}
      mask prompts: Tau "Time Constant"; Ts "Sample Time"
  Bus Creator : BusCreator  Inputs=4
  Compare To Constant : simulink/Logic and Bit Operations/Compare To Constant  relop=>  const=Vdc_max  OutDataTypeStr=boolean
  Constant : Constant  Value=Iac_max
  Debounce : Subsystem  mask{Ts=Ts, Td=5}
      mask prompts: Ts "Sample Time"; Td "Debounce Time"
  Gain : Gain  Gain=1/(VacRMS*sqrt(2))
  Idq_con_disc : Subsystem  mask{L=L, iq_max=Iq_at_max, id_max=Id_at_max*2, kp=I_kp, ki=I_ki, Vdc_nom=Vdc_nom}
      mask prompts: L "Boost Inductor"; iq_max "Maximum Iq"; id_max "Maximum Id"; kp "Proportional Gain"; ki "Integral Gain"; Vdc_nom "Nominal DC Bus Voltage"
      mask init:
      | %global_parameters
  Logical Operator : Logic  Operator=NOT  AllPortsSameDT=off  OutDataTypeStr=boolean
  Logical Operator1 : Logic  AllPortsSameDT=off  OutDataTypeStr=boolean
  Logical Operator2 : Logic  Operator=NOT  AllPortsSameDT=off  OutDataTypeStr=boolean
  Logical Operator3 : Logic  Operator=OR  Inputs=4  AllPortsSameDT=off  OutDataTypeStr=boolean
  Logical Operator4 : Logic  Operator=NOT  AllPortsSameDT=off  OutDataTypeStr=boolean
  Logical Operator5 : Logic  Operator=OR  Inputs=1  AllPortsSameDT=off  OutDataTypeStr=boolean
  Logical Operator6 : Logic  Operator=OR  Inputs=1  AllPortsSameDT=off  OutDataTypeStr=boolean
  Modulator : Subsystem
  PLL_disc : Subsystem  mask{PLL_Kp=PLL_Kp, PLL_Ki=PLL_Ki, PLL_freq_range=0.25, PLL_lock_window=0.1}
      mask prompts: PLL_Kp "Proportional Gain"; PLL_Ki "Integral Gain"; PLL_freq_range "PLL Frequency Range"; PLL_lock_window "PLL Lock Window"
  RMS : powerlib_meascontrol/Measurements/RMS  TrueRMS=on  Freq=60/4  RMSInit=0  Ts=Ts
  RT{1,3..5} (4 alike) : RateTransition
  RT{2,6..7,9..11} (6 alike) : RateTransition  OutPortSampleTime=Td_es_min
  Subsystem : Subsystem
  Subsystem1 : Subsystem
  Vac Limit Test : simulink/Logic and Bit Operations/Interval Test  IntervalClosedRight=on  uplimit=VacRMS_limit_pu(1)*VacRMS  IntervalClosedLeft=on  lowlimit=VacRMS_limit_pu(2)*VacRMS  OutDataTypeStr=boolean
  Windowed Limit : Subsystem
  Iabc : Outport
  Vdc : Outport  Port=2
  PLL_freq : Outport  Port=3
  Iqd : Outport  Port=4
  Faults : Outport  Port=5
  wires:
  Debounce/1(Out) -> Logical Operator2/1
  Logical Operator6/1 -> Logical Operator3/1
  Logical Operator3/1 -> [anyFault]
  Logical Operator2/1 -> Logical Operator1/2
  Break Algebraic Loop/1(Out1) -> Iqd/1, Subsystem/1(qd), RT7/1
  RMS/1 -> Vac Limit Test/1
  Vac Limit Test/1 -> Logical Operator4/1  "ACVoltage"
  Logical Operator4/1 -> Logical Operator5/1
  RT3/1 -> Boost_rectifier_average_model_disc/1, RT9/1
  PLL_disc/1(theta) -> [theta]
  [theta] -> Subsystem/2(theta)
  [theta] -> Subsystem1/2(theta)
  PLL_disc/3(locked) -> [PLL]  "PLL"
  [PLL] -> Logical Operator/1
  [anyFault] -> Debounce/1(In)
  Bus Creator/1 -> Faults/1  "faults"
  Subsystem1/1(qd) -> RT3/1
  Boost_rectifier_average_model_disc/1 -> Break Algebraic Loop/1(In1)
  Subsystem/1(abc) -> Iabc/1, [Iabc]
  Iqd_ref/1 -> RT6/1
  Idq_con_disc/1(Vqd) -> Modulator/1(Vqd)
  idc/1 -> RT4/1
  Logical Operator1/1 -> RT10/1
  Constant/1 -> Windowed Limit/2(Threshold)
  Windowed Limit/1(TestOut) -> Logical Operator6/1, Bus Creator/1  "Iac_Over_Under"
  Compare To Constant/1 -> Logical Operator3/2, Bus Creator/2  "Vdc_Overvoltage"
  PLL_disc/2(freq) -> PLL_freq/1
  Modulator/1(dqd) -> RT1/1
  Logical Operator/1 -> Logical Operator3/3, Bus Creator/3  "PLL_not_locked"
  Gain/1 -> PLL_disc/1(abc)
  Enable/1 -> Logical Operator1/1
  RT1/1 -> Boost_rectifier_average_model_disc/2
  Vabc/1 -> RT2/1, [Vabc]
  RT2/1 -> Gain/1, Subsystem1/1(abc)
  RT4/1 -> Boost_rectifier_average_model_disc/3
  RT5/1 -> Boost_rectifier_average_model_disc/4
  RT6/1 -> Idq_con_disc/1(Iqd_ref)
  RT7/1 -> Idq_con_disc/2(Iqd)
  Boost_rectifier_average_model_disc/2 -> Vdc/1, RT11/1, Compare To Constant/1
  RT9/1 -> Idq_con_disc/3(Vqd_ff)
  RT10/1 -> Idq_con_disc/4(En), RT5/1
  RT11/1 -> Idq_con_disc/5(Vdc), Modulator/2(Vdc)
  Logical Operator5/1 -> Logical Operator3/4, Bus Creator/4  "Vac_Over_Under"
  [Vabc] -> RMS/1
  [Iabc] -> Windowed Limit/1(Signal)

== system PV_lib/PV/PV System/PV ==
  Irradiance : Inport
  Temp : Inport  Port=2
  Vpv : Inport  Port=3
  Bus Creator : BusCreator  Inputs=5
  Controlled Voltage Source : powerlib/Electrical Sources/Controlled Voltage Source  Initialize=on  Source_Type=DC  Amplitude=1200  Phase=0  Frequency=0  Measurements=None
  Diode : Subsystem
      mask Display:
      | plot(-75,-50,100,150, [-15 -15 43 -15 -15 -75],[50 8 50 92 50 50], ...
      |     [43 43],[8 94],[100 43], [50 50])
  Gain1 : Gain  Gain=Rs*Nser/Npar  SaturateOnIntegerOverflow=on  OutDataTypeStr=Inherit: Same as input  ParamDataTypeStr=Inherit: Same as input
  IL : powerlib/Electrical Sources/Controlled Current Source  Initialize=on  Source_Type=AC  Amplitude=0  Phase=0  Frequency=0  Measurements=None
  I_PV : powerlib/Measurements/Current Measurement  PhasorSimulation=off  OutputType=Complex  PSBequivalent=0
  Light current IL : Subsystem
  Product : Product  RndMeth=Zero
  Rs : powerlib/Elements/Series RLC Branch  LConnTagsString=__new0  RConnTagsString=__new0  BranchType=R  Resistance=Rs*Nser/Npar  Inductance=1e-3  SetiL0=off  InitialCurrent=0  Capacitance=1e-6  Setx0=off  InitialVoltage=0  Measurements=None
  Rsh : powerlib/Elements/Series RLC Branch  LConnTagsString=__new0  RConnTagsString=__new0  BranchType=R  Resistance=Rsh*Nser/Npar  Inductance=1e-3  SetiL0=off  InitialCurrent=0  Capacitance=1e-6  Setx0=off  InitialVoltage=0  Measurements=Branch current
  Sum2 : Sum  SaturateOnIntegerOverflow=on  InputSameDT=on  OutDataTypeStr=Inherit: Same as first input
  V_PV : powerlib/Measurements/Voltage Measurement  PhasorSimulation=off  OutputType=Complex  PSBequivalent=0
  m : Outport
  Ipv : Outport  Port=2
  wires:
  Light current IL/2(Tcell_K) -> Diode/2(Tcell_K)
  Vpv/1 -> Controlled Voltage Source/1
  Irradiance/1 -> Light current IL/2(Irradiance), Bus Creator/5  "Irradiance (W/m^2)"
  Light current IL/1(IL) -> IL/1
  V_PV/1 -> Sum2/2, Bus Creator/1, Product/1  "V_PV"
  I_PV/1 -> Ipv/1, Gain1/1, Bus Creator/2, Product/2  "I_PV"
  Sum2/1 -> Diode/1(Vd)
  Gain1/1 -> Sum2/1
  Temp/1 -> Light current IL/1(Temperature), Bus Creator/4  "Temperature (C)"
  Bus Creator/1 -> m/1
  Product/1 -> Bus Creator/3  "P_PV"
  connections:
  Rsh/LConn1 -- Diode/LConn1 -- IL/RConn1 -- Rs/RConn1
  V_PV/LConn2 -- Controlled Voltage Source/LConn1 -- Rsh/RConn1 -- IL/LConn1 -- Diode/RConn1
  Rs/LConn1 -- I_PV/LConn1
  V_PV/LConn1 -- I_PV/RConn1 -- Controlled Voltage Source/RConn1

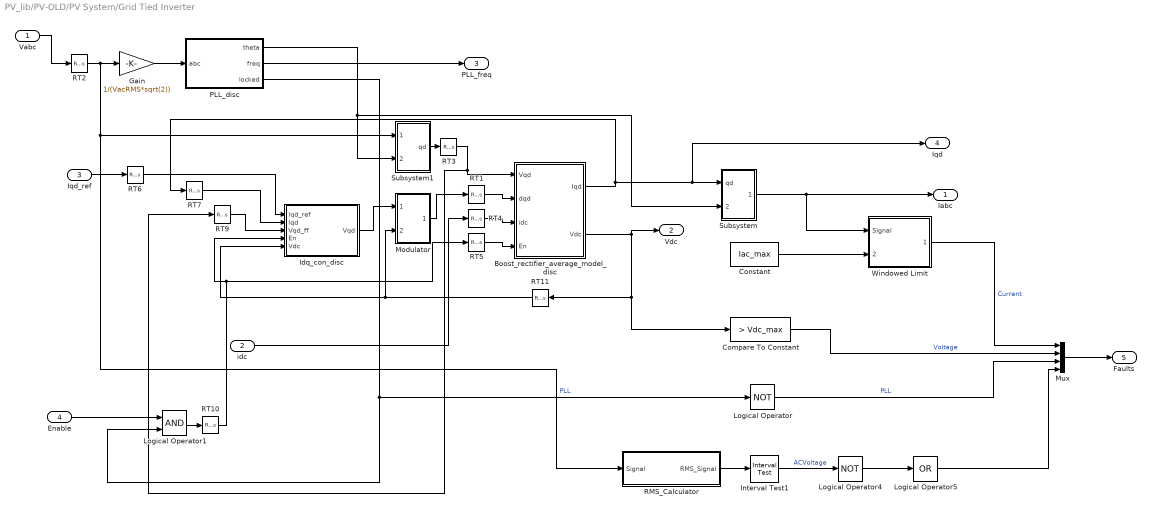
== system PV_lib/PV-OLD/PV System/Grid Tied Inverter ==
  Vabc : Inport
  idc : Inport  Port=2
  Iqd_ref : Inport  Port=3
  Enable : Inport  Port=4
  Boost_rectifier_average_model_disc : Subsystem  mask{C=C, L=L, Roff=Roff, Vdc_nom=Vdc_nom}
      mask prompts: C "DC Bus Capacitance"; L "Boost Inductor"; Roff "Switch resistance when off"; Vdc_nom "Nominal DC Bus Voltage"
      mask init:
      | global_parameters
  Compare To Constant : simulink/Logic and Bit Operations/Compare To Constant  relop=>  const=Vdc_max  OutDataTypeStr=boolean
  Constant : Constant  Value=Iac_max
  Gain : Gain  Gain=1/(VacRMS*sqrt(2))
  Idq_con_disc : Subsystem  mask{L=L, iq_max=Iq_at_max, id_max=Id_at_max*2, kp=I_kp, ki=I_ki, Vdc_nom=Vdc_nom}
      mask prompts: L "Boost Inductor"; iq_max "Maximum Iq"; id_max "Maximum Id"; kp "Proportional Gain"; ki "Integral Gain"; Vdc_nom "Nominal DC Bus Voltage"
      mask init:
      | global_parameters
  Interval Test1 : simulink/Logic and Bit Operations/Interval Test  IntervalClosedRight=on  uplimit=VacRMS*1.1  IntervalClosedLeft=on  lowlimit=VacRMS*0.9  OutDataTypeStr=boolean
  Logical Operator : Logic  Operator=NOT  AllPortsSameDT=off  OutDataTypeStr=boolean
  Logical Operator1 : Logic  AllPortsSameDT=off  OutDataTypeStr=boolean
  Logical Operator4 : Logic  Operator=NOT  AllPortsSameDT=off  OutDataTypeStr=boolean
  Logical Operator5 : Logic  Operator=OR  Inputs=1  AllPortsSameDT=off  OutDataTypeStr=boolean
  Modulator : Subsystem
  Mux : Mux
  PLL_disc : Subsystem  mask{PLL_Kp=PLL_Kp, PLL_Ki=PLL_Ki, PLL_freq_range=0.25, PLL_lock_window=0.1}
      mask prompts: PLL_Kp "Proportional Gain"; PLL_Ki "Integral Gain"; PLL_freq_range "PLL Frequency Range"; PLL_lock_window "PLL Lock Window"
  RMS_Calculator : Subsystem
  RT{1,3..5} (4 alike) : RateTransition
  RT{2,6..7,9..11} (6 alike) : RateTransition  OutPortSampleTime=Td_es_min
  Subsystem : Subsystem
  Subsystem1 : Subsystem
  Windowed Limit : Subsystem
  Iabc : Outport
  Vdc : Outport  Port=2
  PLL_freq : Outport  Port=3
  Iqd : Outport  Port=4
  Faults : Outport  Port=5
  wires:
  RT11/1 -> Modulator/2(Vdc), Idq_con_disc/5(Vdc)
  RT10/1 -> RT5/1, Idq_con_disc/4(En)
  RT9/1 -> Idq_con_disc/3(Vqd_ff)
  Boost_rectifier_average_model_disc/2(Vdc) -> Compare To Constant/1, RT11/1, Vdc/1
  RT7/1 -> Idq_con_disc/2(Iqd)
  RT6/1 -> Idq_con_disc/1(Iqd_ref)
  RT5/1 -> Boost_rectifier_average_model_disc/4(En)
  RT4/1 -> Boost_rectifier_average_model_disc/3(idc)
  RT3/1 -> RT9/1, Boost_rectifier_average_model_disc/1(Vqd)
  RT2/1 -> Gain/1, Subsystem1/1(abc), RMS_Calculator/1(Signal)
  Vabc/1 -> RT2/1
  RT1/1 -> Boost_rectifier_average_model_disc/2(dqd)
  PLL_disc/1(theta) -> Subsystem1/2(theta), Subsystem/2(theta)
  Enable/1 -> Logical Operator1/1
  Gain/1 -> PLL_disc/1(abc)
  Logical Operator/1 -> Mux/3  "PLL"
  PLL_disc/3(locked) -> Logical Operator1/2, Logical Operator/1  "PLL"
  Modulator/1(dqd) -> RT1/1
  PLL_disc/2(freq) -> PLL_freq/1
  Compare To Constant/1 -> Mux/2  "Voltage"
  Windowed Limit/1(TestOut) -> Mux/1  "Current"
  Constant/1 -> Windowed Limit/2(Threshold)
  Logical Operator1/1 -> RT10/1
  idc/1 -> RT4/1
  Idq_con_disc/1(Vqd) -> Modulator/1(Vqd)
  Iqd_ref/1 -> RT6/1
  Subsystem/1(abc) -> Iabc/1, Windowed Limit/1(Signal)
  Boost_rectifier_average_model_disc/1(Iqd) -> RT7/1, Iqd/1, Subsystem/1(qd)
  Subsystem1/1(qd) -> RT3/1
  Mux/1 -> Faults/1
  Logical Operator4/1 -> Logical Operator5/1
  Interval Test1/1 -> Logical Operator4/1  "ACVoltage"
  RMS_Calculator/1(RMS_Signal) -> Interval Test1/1
  Logical Operator5/1 -> Mux/4

== system PV_lib/PV-OLD/PV System/PV ==
  Irradiance : Inport
  Temp : Inport  Port=2
  Vpv : Inport  Port=3
  Bus Creator : BusCreator  Inputs=5
  Controlled Voltage Source : powerlib/Electrical Sources/Controlled Voltage Source  Initialize=on  Source_Type=DC  Amplitude=1200  Phase=0  Frequency=0  Measurements=None
  Diode : Subsystem
      mask Display:
      | plot(-75,-50,100,150, [-15 -15 43 -15 -15 -75],[50 8 50 92 50 50], ...
      |     [43 43],[8 94],[100 43], [50 50])
  Gain1 : Gain  Gain=Rs*Nser/Npar  SaturateOnIntegerOverflow=on  OutDataTypeStr=Inherit: Same as input  ParamDataTypeStr=Inherit: Same as input
  IL : powerlib/Electrical Sources/Controlled Current Source  Initialize=on  Source_Type=AC  Amplitude=0  Phase=0  Frequency=0  Measurements=None
  I_PV : powerlib/Measurements/Current Measurement  PhasorSimulation=off  OutputType=Complex  PSBequivalent=0
  Light current IL : Subsystem
  Product : Product  RndMeth=Zero
  Rs : powerlib/Elements/Series RLC Branch  LConnTagsString=__new0  RConnTagsString=__new0  BranchType=R  Resistance=Rs*Nser/Npar  Inductance=1e-3  SetiL0=off  InitialCurrent=0  Capacitance=1e-6  Setx0=off  InitialVoltage=0  Measurements=None
  Rsh : powerlib/Elements/Series RLC Branch  LConnTagsString=__new0  RConnTagsString=__new0  BranchType=R  Resistance=Rsh*Nser/Npar  Inductance=1e-3  SetiL0=off  InitialCurrent=0  Capacitance=1e-6  Setx0=off  InitialVoltage=0  Measurements=Branch current
  Sum2 : Sum  SaturateOnIntegerOverflow=on  InputSameDT=on  OutDataTypeStr=Inherit: Same as first input
  V_PV : powerlib/Measurements/Voltage Measurement  PhasorSimulation=off  OutputType=Complex  PSBequivalent=0
  m : Outport
  Ipv : Outport  Port=2
  wires:
  Product/1 -> Bus Creator/3  "P_PV"
  Bus Creator/1 -> m/1
  Temp/1 -> Bus Creator/4, Light current IL/1(Temperature)  "Temperature (C)"
  Gain1/1 -> Sum2/1
  Sum2/1 -> Diode/1(Vd)
  I_PV/1 -> Product/2, Bus Creator/2, Gain1/1, Ipv/1  "I_PV"
  V_PV/1 -> Product/1, Bus Creator/1, Sum2/2  "V_PV"
  Light current IL/1(IL) -> IL/1
  Irradiance/1 -> Bus Creator/5, Light current IL/2(Irradiance)  "Irradiance (W/m^2)"
  Vpv/1 -> Controlled Voltage Source/1
  Light current IL/2(Tcell_K) -> Diode/2(Tcell_K)
  connections:
  Controlled Voltage Source/RConn1 -- I_PV/RConn1 -- V_PV/LConn1
  Rs/LConn1 -- I_PV/LConn1
  Diode/RConn1 -- IL/LConn1 -- Rsh/RConn1 -- Controlled Voltage Source/LConn1 -- V_PV/LConn2
  Rs/RConn1 -- IL/RConn1 -- Diode/LConn1 -- Rsh/LConn1

== system PV_lib/PV/PV System/Grid Tied Inverter/Break Algebraic Loop ==
  In1 : Inport
  1/Tr : Gain  Gain=1/Tau  SampleTime=Ts
  Discrete-Time Integrator : DiscreteIntegrator  SampleTime=Ts  ICPrevOutput=DiscIntNeverNeededParam  ICPrevScaledInput=DiscIntNeverNeededParam
  Sum : Sum  Inputs=|+-
  Out1 : Outport
  wires:
  Sum/1 -> 1/Tr/1
  1/Tr/1 -> Discrete-Time Integrator/1
  Discrete-Time Integrator/1 -> Sum/2, Out1/1
  In1/1 -> Sum/1

== system PV_lib/PV/PV System/Grid Tied Inverter/Debounce ==
  In : Inport
  Compare To Constant1 : simulink/Logic and Bit Operations/Compare To Constant  relop=>  const=1  OutDataTypeStr=boolean
  Discrete-Time Integrator : DiscreteIntegrator  IntegratorMethod=Accumulation: Forward Euler  gainval=Ts/Td  ExternalReset=level  SampleTime=Ts  OutDataTypeStr=double  UpperSaturationLimit=1.001  LowerSaturationLimit=0  ICPrevOutput=DiscIntNeverNeededParam  ICPrevScaledInput=DiscIntNeverNeededParam
  Logical Operator : Logic  Operator=NOT  AllPortsSameDT=off  OutDataTypeStr=boolean
  Out : Outport
  wires:
  Discrete-Time Integrator/1 -> Compare To Constant1/1
  Logical Operator/1 -> Discrete-Time Integrator/2
  In/1 -> Discrete-Time Integrator/1, Logical Operator/1
  Compare To Constant1/1 -> Out/1
